simulink model "W07_E_notch"  (R2024b)
settings: Solver=ode4  StartTime=0  StopTime=T_final  FixedStep=h  RelTol=1e-3
values from neighbouring files (symbols this model uses):
  beta_c = pi/2    (= 1.57079632679)    [W07_0_setup.m]
  k_neg = cfg.k_neg    [W07_0_setup.m]
  k_pos = cfg.k_pos    [W07_0_setup.m]
  Kd = 100    [W07_0_setup.m]
  Kp = 300    [W07_0_setup.m]
  mp = 25    [W07_0_setup.m]
  N_max = min(2*cfg.y_pont*(cfg.k_pos*cfg.n_max^2 - X_ff/2),              2*cfg.y_pont*(X_ff/2 + cfg.k_neg*cfg.n_min^2))    [W07_0_setup.m]
  psi_step = 10    [W07_0_setup.m]
  rp = [0.05 0 -0.35]'    [W07_0_setup.m]
  T_max = cfg.k_pos*cfg.n_max^2    [W07_0_setup.m]
  T_min = -cfg.k_neg*cfg.n_min^2    [W07_0_setup.m]
  t_step = 5    [W07_0_setup.m]
  V_c = 0    [W07_0_setup.m]
  w0 = 2*pi/T0    (= 3.14159265359)    [W07_0_setup.m]    (also in W07_C_sea_as_signal.m = 2 pi / T0 =)
  wave_on = 1    [W07_0_setup.m]
  x0 = zeros(12,1)    [W07_0_setup.m]
  X_ff = 60    [W07_0_setup.m]
  y_pont = cfg.y_pont    [W07_0_setup.m]
  zeta_d = 0.3    [W07_0_setup.m]
  zeta_n = 0.05    [W07_0_setup.m]
undefined symbols (not defined in the file or in its folder): a_i, k_w, phi_i, w_i
settings Model: Creator=admin  LastModifiedBy=admin
settings DataIOCC: ReturnWorkspaceOutputs=off

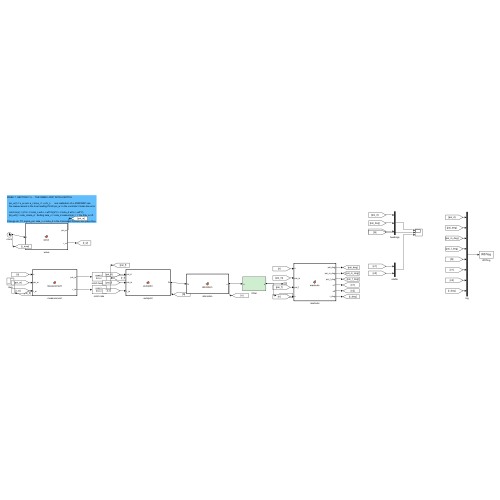
[thumbnail: Simulink's stored preview of the top-level diagram]
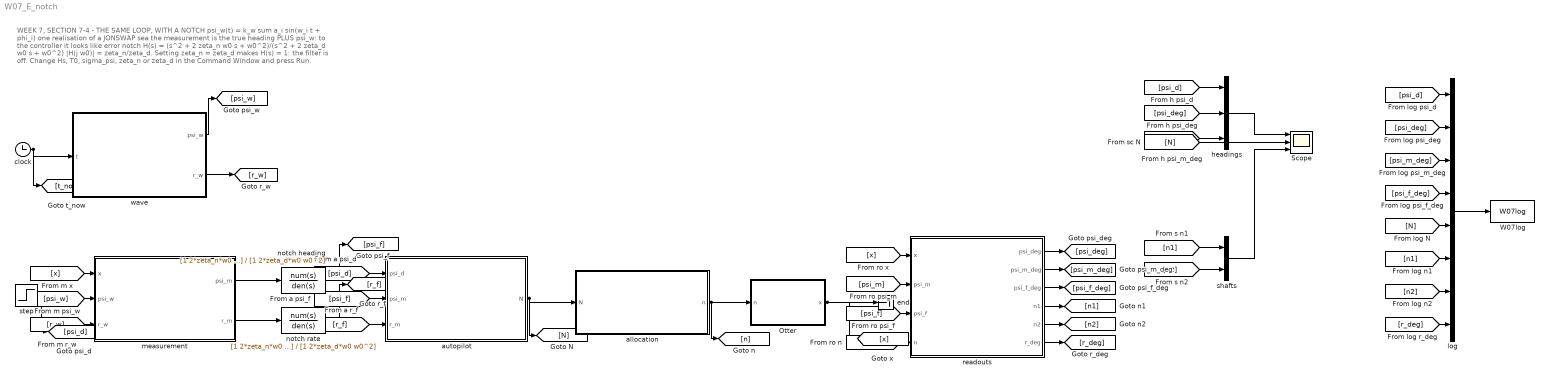
== system W07_E_notch ==
  note: WEEK 7, SECTION 7-4  -  THE SAME LOOP, WITH A NOTCH
      |
      |    psi_w(t) = k_w sum a_i sin(w_i t + phi_i)      one realisation of a JONSWAP sea
      |    the measurement is the true heading PLUS psi_w: to the controller it looks like error
      |
      |    notch H(s) = (s^2 + 2 zeta_n w0 s + w0^2)/(s^2 + 2 zeta_d w0 s + w0^2)
      |    |H(j w0)| = zeta_n/zeta_d.  Setting zeta_n = zeta_d makes H(s) = 1: the filter is off.
      |
      | Change Hs, T0, sigma_psi, zeta_n or zeta_d in the Command Window and press Run.
  Otter : Subsystem
  Scope : Scope  NumInputPorts=3
  W07log : ToWorkspace  VariableName=W07log  SaveFormat=Structure With Time  SampleTime=-1
  allocation : MATLAB Function  TreatAsAtomicUnit=on
  autopilot : MATLAB Function  TreatAsAtomicUnit=on
  clock : Clock
  end : Terminator
  headings : Mux  Inputs=3
  log : Mux  Inputs=8
  measurement : MATLAB Function  TreatAsAtomicUnit=on
  notch heading : TransferFcn  Numerator=[1 2*zeta_n*w0 w0^2]  Denominator=[1 2*zeta_d*w0 w0^2]
  notch rate : TransferFcn  Numerator=[1 2*zeta_n*w0 w0^2]  Denominator=[1 2*zeta_d*w0 w0^2]
  readouts : MATLAB Function  TreatAsAtomicUnit=on
  shafts : Mux  Inputs=2
  step : Step  Time=t_step  After=psi_step  SampleTime=0
  wave : MATLAB Function  TreatAsAtomicUnit=on
  wires:
  clock/1 -> wave/1(t), [t_now]
  wave/1(psi_w) -> [psi_w]
  wave/2(r_w) -> [r_w]
  step/1 -> [psi_d]
  [x] -> measurement/1(x)
  [psi_w] -> measurement/2(psi_w)
  [r_w] -> measurement/3(r_w)
  measurement/1(psi_m) -> notch heading/1
  notch heading/1 -> [psi_f]
  measurement/2(r_m) -> notch rate/1
  notch rate/1 -> [r_f]
  [psi_d] -> autopilot/1(psi_d)
  [psi_f] -> autopilot/2(psi_m)
  [r_f] -> autopilot/3(r_m)
  autopilot/1(N) -> [N], allocation/1(N)
  allocation/1(n) -> [n], Otter/1(n)
  Otter/1(x) -> [x], end/1
  [x] -> readouts/1(x)
  [psi_m] -> readouts/2(psi_m)
  [psi_f] -> readouts/3(psi_f)
  [n] -> readouts/4(n)
  readouts/1(psi_deg) -> [psi_deg]
  readouts/2(psi_m_deg) -> [psi_m_deg]
  readouts/3(psi_f_deg) -> [psi_f_deg]
  readouts/4(n1) -> [n1]
  readouts/5(n2) -> [n2]
  readouts/6(r_deg) -> [r_deg]
  [psi_d] -> headings/1
  [psi_deg] -> headings/2
  [psi_m_deg] -> headings/3
  headings/1 -> Scope/1
  [N] -> Scope/2
  [n1] -> shafts/1
  [n2] -> shafts/2
  shafts/1 -> Scope/3
  [psi_d] -> log/1
  [psi_deg] -> log/2
  [psi_m_deg] -> log/3
  [psi_f_deg] -> log/4
  [N] -> log/5
  [n1] -> log/6
  [n2] -> log/7
  [r_deg] -> log/8
  log/1 -> W07log/1

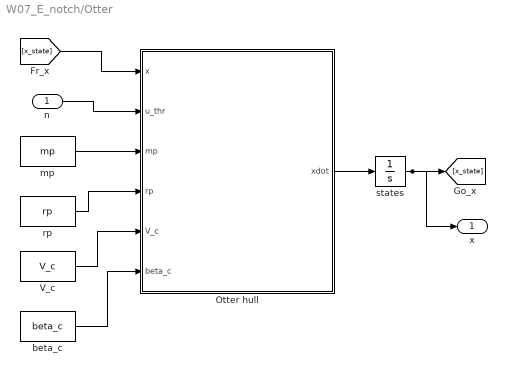
== system W07_E_notch/Otter ==
  n : Inport
  Otter hull : MATLAB Function  TreatAsAtomicUnit=on
  V_c : Constant  Value=V_c
  beta_c : Constant  Value=beta_c
  mp : Constant  Value=mp
  rp : Constant  Value=rp
  states : Integrator  InitialCondition=x0
  x : Outport
  wires:
  n/1 -> Otter hull/2(u_thr)
  [x_state] -> Otter hull/1(x)
  mp/1 -> Otter hull/3(mp)
  rp/1 -> Otter hull/4(rp)
  V_c/1 -> Otter hull/5(V_c)
  Otter hull/1(xdot) -> states/1
  beta_c/1 -> Otter hull/6(beta_c)
  states/1 -> [x_state], x/1

== matlab function W07_E_notch/measurement ==
  data: x input; psi_m output double size=[1 1]; psi_w input; r_w input; r_m output
function [psi_m, r_m] = measurement(x, psi_w, r_w)
%#codegen
%  제어기가 보는 것 = 배가 실제로 하는 것 + 1차 파랑
%  What the controller sees = what the vessel really does + the first-order wave
%
%  배는 파랑을 따라 흔들리고 센서는 그것을 정직하게 잰다. 제어기에게는 그 흔들림이
%  **오차**로 보인다 — 그것이 이번 주가 다루는 상황이다.
%  The vessel oscillates with the sea and the sensor reports it truthfully; to the
%  controller that oscillation looks like error, which is the subject of this week.
psi_m = x(12)*180/pi + psi_w;    % [deg]
r_m   = x(6)*180/pi  + r_w;      % [deg/s]

== matlab function W07_E_notch/wave ==
  data: t input; psi_w output double size=[1 1]; r_w output; w_i parameter; a_i parameter; phi_i parameter; k_w parameter; wave_on parameter
function [psi_w, r_w] = wave(t, w_i, a_i, phi_i, k_w, wave_on)
%#codegen
%  1차 파랑이 만드는 선수각과 그 변화율 / the wave-induced heading and its rate
%
%  스펙트럼 하나를 성분 여럿의 합으로 적는다. 진폭은 JONSWAP 에서 나오고 (wave_train),
%  위상은 정해져 있으므로 이 바다는 매번 똑같다 — 강의의 표를 재현할 수 있다.
%  One spectrum, written as a sum of components: the amplitudes come from JONSWAP
%  and the phases are fixed, so this sea is the same on every run.
%
%      psi_w(t) = k_w * sum_i a_i sin(w_i t + phi_i)          [deg]
%      r_w(t)   = k_w * sum_i a_i w_i cos(w_i t + phi_i)      [deg/s]
%
%  k_w 는 진폭 [m] 을 선수각 [deg] 으로 바꾸는 배율이다. 이 주차는 그 응답을
%  유도하지 않고 **주어진 것으로** 둔다 — 표준편차 sigma_psi 로 적는다.
%  k_w turns a wave amplitude into a heading. This week does not derive that
%  response; it takes it as given, stated by its standard deviation.
psi_w = 0;  r_w = 0;
if wave_on ~= 0
    for i = 1:numel(w_i)
        psi_w = psi_w + k_w*a_i(i)*sin(w_i(i)*t + phi_i(i));
        r_w   = r_w   + k_w*a_i(i)*w_i(i)*cos(w_i(i)*t + phi_i(i));
    end
end

== matlab function W07_E_notch/autopilot ==
  settings: updateMethod=DISCRETE  sampleTime=h
  data: psi_d input; N output double size=[1 1]; psi_m input; r_m input; Kp parameter; Kd parameter; N_max parameter
function N = autopilot(psi_d, psi_m, r_m, Kp, Kd, N_max)
%#codegen
%  4주차의 오토파일럿. 게인은 그대로다 — 바뀐 것은 계측뿐이다.
%  The Week 4 autopilot, gains unchanged; only the measurement is different.
%
%      N = Kp ssa(psi_d - psi_m) - Kd r_m,   |N| <= N_max
e = (psi_d - psi_m)*pi/180;
e = atan2(sin(e), cos(e));            % 감김 / the wrap of Week 4
u = Kp*e - Kd*r_m*pi/180;
N = min(max(u, -N_max), N_max);

== matlab function W07_E_notch/allocation ==
  data: N input; n output double size=[2 1]; X_ff parameter; y_pont parameter; k_pos parameter; k_neg parameter; T_max parameter; T_min parameter
function n = allocation(N, X_ff, y_pont, k_pos, k_neg, T_max, T_min)
%#codegen
%  6주차의 배분: 정사각 규칙, 비율로 줄이기, 그리고 곡선의 역
%  The allocation of Week 6: the square rule, scaling, and the inverse curve
T1 = X_ff/2 + N/(2*y_pont);
T2 = X_ff/2 - N/(2*y_pont);
s = 1;
if T1 > T_max, s = min(s, T_max/T1); end
if T2 > T_max, s = min(s, T_max/T2); end
if T1 < T_min, s = min(s, T_min/T1); end
if T2 < T_min, s = min(s, T_min/T2); end
T1 = s*T1;  T2 = s*T2;
k1 = k_pos;  if T1 < 0, k1 = k_neg; end
k2 = k_pos;  if T2 < 0, k2 = k_neg; end
n = [sign(T1)*sqrt(abs(T1)/k1); sign(T2)*sqrt(abs(T2)/k2)];

== matlab function W07_E_notch/Otter/Otter hull ==
  data: x input; xdot output double size=[12 1]; u_thr input; mp input; rp input; V_c input; beta_c input
function xdot = otter_hull(x, u_thr, mp, rp, V_c, beta_c)
% Fossen's otter.m, called unchanged from Tools/MSS/VESSELS.
%
%   x       12 states, fed back from the integrator
%   u_thr   propeller shaft speeds [rad/s]
%
% otter.m is not written for code generation, so the call is extrinsic and
% xdot has to be pre-sized for Simulink to know the output width.
coder.extrinsic('otter');

xdot = zeros(12,1);
xdot = otter(x, u_thr, mp, rp, V_c, beta_c);
end

== matlab function W07_E_notch/readouts ==
  data: x input; psi_deg output double size=[1 1]; psi_m input; psi_f input; n input; psi_m_deg output; psi_f_deg output; n1 output; n2 output; r_deg output
function [psi_deg, psi_m_deg, psi_f_deg, n1, n2, r_deg] = readouts(x, psi_m, psi_f, n)
%#codegen
%  표시와 기록만 한다 / display and logging only
psi_deg   = x(12)*180/pi;    % 배의 진짜 선수각 / the true heading
psi_m_deg = psi_m;           % 계측값 (진짜 + 파랑) / the measurement
psi_f_deg = psi_f;           % 제어기가 쓰는 값 / what the controller uses
n1 = n(1);  n2 = n(2);
r_deg = x(6)*180/pi;
